simulink model "simulink"  (R2024a)
settings: Solver=ode2  StartTime=0.0  StopTime=100  FixedStep=0.08  RelTol=1e-3  EnableMultiTasking=on
settings Model: Creator=baron  LastModifiedBy=ngoba
settings SolverCC: AlgebraicLoopSolver=TrustRegion
settings DebuggingCC: UnconnectedInputMsg=warning  UnconnectedOutputMsg=warning  UnconnectedLineMsg=warning
settings ModelReferenceCC: EnableRefExpFcnMdlSchedulingChecks=on
settings RTWCC: GPUComputeCapability=3.5

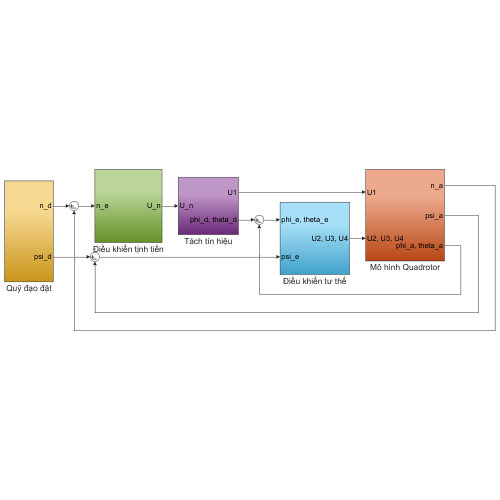
[thumbnail: Simulink's stored preview of the top-level diagram]
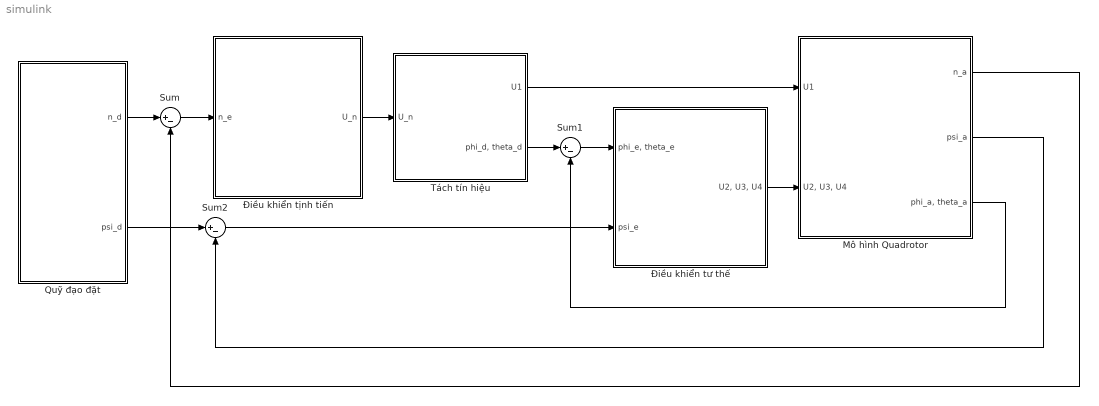
== system simulink ==
  Mô hình Quadrotor : Subsystem
  Quỹ đạo đặt : Subsystem
  Sum : Sum  Inputs=|+-
  Sum1 : Sum  Inputs=|+-
  Sum2 : Sum  Inputs=|+-
  Tách tín hiệu : Subsystem
  Điều khiển tư thế : Subsystem
  Điều khiển tịnh tiến : Subsystem
  wires:
  Sum/1 -> Điều khiển tịnh tiến/1(n_e)
  Quỹ đạo đặt/1(n_d) -> Sum/1
  Điều khiển tịnh tiến/1(U_n) -> Tách tín hiệu/1(U_n)
  Sum1/1 -> Điều khiển tư thế/1("phi_e, theta_e")
  Sum2/1 -> Điều khiển tư thế/2(psi_e)
  Mô hình Quadrotor/1(n_a) -> Sum/2
  Mô hình Quadrotor/2(psi_a) -> Sum2/2
  Mô hình Quadrotor/3("phi_a, theta_a") -> Sum1/2
  Tách tín hiệu/1(U1) -> Mô hình Quadrotor/1(U1)
  Tách tín hiệu/2("phi_d, theta_d") -> Sum1/1
  Điều khiển tư thế/1("U2, U3, U4") -> Mô hình Quadrotor/2("U2, U3, U4")
  Quỹ đạo đặt/2(psi_d) -> Sum2/1

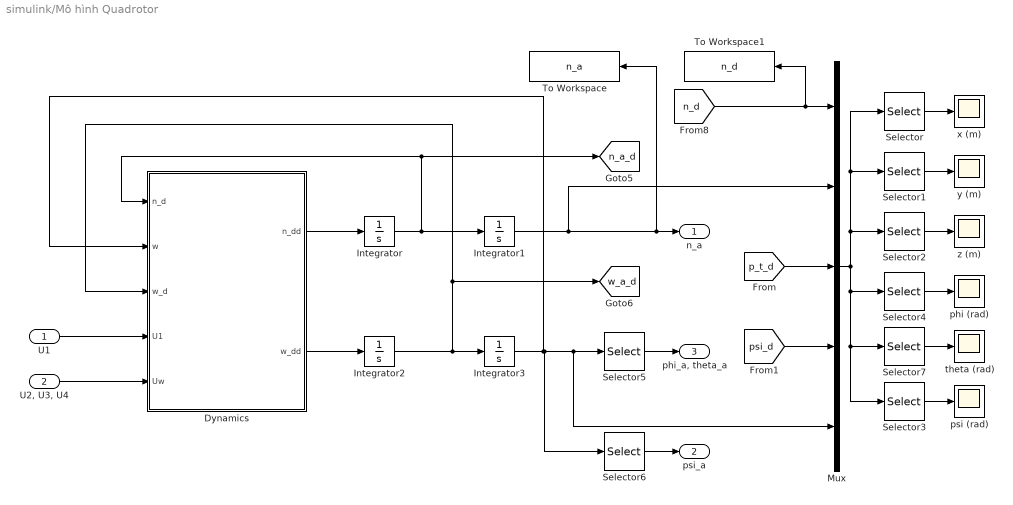
== system simulink/Mô hình Quadrotor ==
  U1 : Inport
  "U2, U3, U4" : Inport  Port=2
  Dynamics : MATLAB Function  TreatAsAtomicUnit=on
  Integrator{,1..3} (4 alike) : Integrator  InitialCondition=[0, 0, 0]'
  Mux : Mux  Inputs=5
  Selector : Selector  InputPortWidth=12  IndexOptions=Index vector (dialog)  Indices=[4 1]  OutputSizes=1
  Selector1 : Selector  InputPortWidth=12  IndexOptions=Index vector (dialog)  Indices=[5 2]  OutputSizes=1
  Selector2 : Selector  InputPortWidth=12  IndexOptions=Index vector (dialog)  Indices=[6 3]  OutputSizes=1
  Selector3 : Selector  InputPortWidth=12  IndexOptions=Index vector (dialog)  Indices=[12 9]  OutputSizes=1
  Selector4 : Selector  InputPortWidth=12  IndexOptions=Index vector (dialog)  Indices=[10 7]  OutputSizes=1
  Selector5 : Selector  InputPortWidth=3  IndexOptions=Index vector (dialog)  Indices=[1 2]  OutputSizes=1
  Selector6 : Selector  InputPortWidth=3  IndexOptions=Index vector (dialog)  Indices=[3]  OutputSizes=1
  Selector7 : Selector  InputPortWidth=12  IndexOptions=Index vector (dialog)  Indices=[11 8]  OutputSizes=1
  To Workspace : ToWorkspace  VariableName=n_a  SampleTime=-1
  To Workspace1 : ToWorkspace  VariableName=n_d  SampleTime=-1
  phi (rad) : Scope
  psi (rad) : Scope
  theta (rad) : Scope
  x (m) : Scope
  y (m) : Scope
  z (m) : Scope
  n_a : Outport
  psi_a : Outport  Port=2
  "phi_a, theta_a" : Outport  Port=3
  tag scope: n_a_d=global, w_a_d=global
  wires:
  Integrator/1 -> Integrator1/1, Dynamics/1(n_d), [n_a_d]
  Integrator3/1 -> Selector6/1, Mux/5, Selector5/1, Dynamics/2(w)
  U1/1 -> Dynamics/4(U1)
  Dynamics/1(n_dd) -> Integrator/1
  Dynamics/2(w_dd) -> Integrator2/1
  "U2, U3, U4"/1 -> Dynamics/5(Uw)
  Integrator2/1 -> Integrator3/1, Dynamics/3(w_d), [w_a_d]
  Selector/1 -> x (m)/1
  [n_d] -> To Workspace1/1, Mux/1
  Selector3/1 -> psi (rad)/1
  Selector1/1 -> y (m)/1
  Selector2/1 -> z (m)/1
  Mux/1 -> Selector2/1, Selector1/1, Selector/1, Selector4/1, Selector7/1, Selector3/1
  Integrator1/1 -> Mux/2, To Workspace/1, n_a/1
  Selector6/1 -> psi_a/1
  Selector5/1 -> "phi_a, theta_a"/1
  Selector4/1 -> phi (rad)/1
  Selector7/1 -> theta (rad)/1
  [p_t_d] -> Mux/3
  [psi_d] -> Mux/4

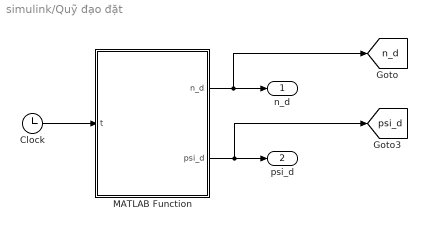
== system simulink/Quỹ đạo đặt ==
  Clock : Clock
  MATLAB Function : MATLAB Function  TreatAsAtomicUnit=on
  n_d : Outport
  psi_d : Outport  Port=2
  tag scope: n_d=global, psi_d=global
  wires:
  Clock/1 -> MATLAB Function/1(t)
  MATLAB Function/1(n_d) -> [n_d], n_d/1
  MATLAB Function/2(psi_d) -> [psi_d], psi_d/1

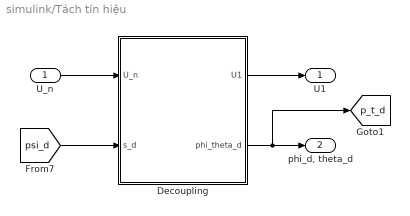
== system simulink/Tách tín hiệu ==
  U_n : Inport
  Decoupling : MATLAB Function  TreatAsAtomicUnit=on
  U1 : Outport
  "phi_d, theta_d" : Outport  Port=2
  tag scope: p_t_d=global
  wires:
  Decoupling/1(U1) -> U1/1
  [psi_d] -> Decoupling/2(s_d)
  U_n/1 -> Decoupling/1(U_n)
  Decoupling/2(phi_theta_d) -> [p_t_d], "phi_d, theta_d"/1

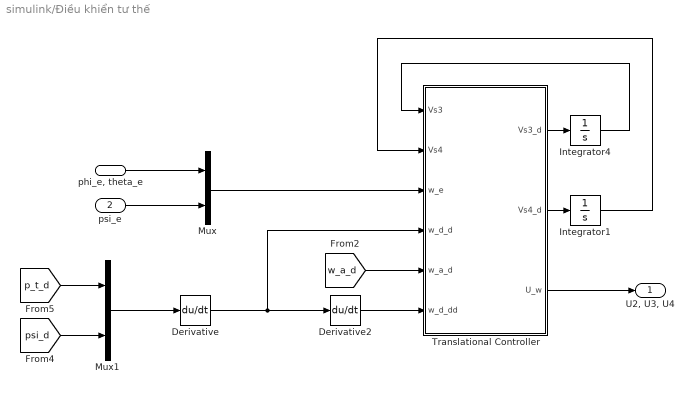
== system simulink/Điều khiển tư thế ==
  "phi_e, theta_e" : Inport
  psi_e : Inport  Port=2
  Derivative : Derivative
  Derivative2 : Derivative
  Integrator1 : Integrator  InitialCondition=[0, 0, 0]'
  Integrator4 : Integrator  InitialCondition=[0, 0, 0]'
  Mux : Mux  Inputs=2
  Mux1 : Mux  Inputs=2
  Translational Controller : MATLAB Function  TreatAsAtomicUnit=on
  "U2, U3, U4" : Outport
  wires:
  Translational Controller/2(Vs4_d) -> Integrator1/1
  Translational Controller/1(Vs3_d) -> Integrator4/1
  [w_a_d] -> Translational Controller/5(w_a_d)
  Derivative2/1 -> Translational Controller/6(w_d_dd)
  Integrator1/1 -> Translational Controller/2(Vs4)
  Translational Controller/3(U_w) -> "U2, U3, U4"/1
  Derivative/1 -> Derivative2/1, Translational Controller/4(w_d_d)
  Integrator4/1 -> Translational Controller/1(Vs3)
  "phi_e, theta_e"/1 -> Mux/1
  psi_e/1 -> Mux/2
  Mux/1 -> Translational Controller/3(w_e)
  Mux1/1 -> Derivative/1
  [psi_d] -> Mux1/2
  [p_t_d] -> Mux1/1

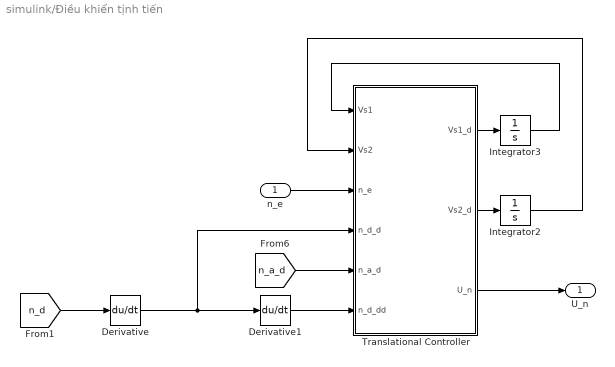
== system simulink/Điều khiển tịnh tiến ==
  n_e : Inport
  Derivative : Derivative
  Derivative1 : Derivative
  Integrator2 : Integrator  InitialCondition=[0, 0, 0]'
  Integrator3 : Integrator  InitialCondition=[0, 0, 0]'
  Translational Controller : MATLAB Function  TreatAsAtomicUnit=on
  U_n : Outport
  wires:
  [n_d] -> Derivative/1
  Derivative/1 -> Translational Controller/4(n_d_d), Derivative1/1
  Translational Controller/3(U_n) -> U_n/1
  Translational Controller/1(Vs1_d) -> Integrator3/1
  Integrator3/1 -> Translational Controller/1(Vs1)
  Translational Controller/2(Vs2_d) -> Integrator2/1
  Integrator2/1 -> Translational Controller/2(Vs2)
  n_e/1 -> Translational Controller/3(n_e)
  Derivative1/1 -> Translational Controller/6(n_d_dd)
  [n_a_d] -> Translational Controller/5(n_a_d)

== matlab function simulink/Mô hình Quadrotor/Dynamics ==
  settings: updateMethod=DISCRETE
  data: n_d input; n_dd output; w_dd output; w input; w_d input; U1 input; Uw input
function [n_dd, w_dd] = fcn(n_d, w, w_d, U1, Uw)
    % Parameters
    m = 0.486;
    g = 9.810;
    Mm = diag([m, m, m]);
    Gg = [0, 0, -m*g]';
    l = diag([0.250, 0.250, 1]);
    I = diag([4.856e-3, 4.856e-3, 8.801e-3]);
    cdn = diag([5.560e-4, 5.560e-4, 6.350e-4]);
    kdn = diag([1e-4, 1e-4, 1e-4]);
    kp = 3.230e-7;
    kd = 2.980e-5;
    W_to_U = [ kd,  kd, kd,  kd;
                0,  kd,  0, -kd;
              -kd,   0, kd,   0;
               kp, -kp, kp, -kp];
    Ir = diag([5e-5, 5e-5, 5e-5]);
    % Translational function
    FD = -cdn*n_d;   
    % Rotational function
    W = sqrt((W_to_U^-1)*[U1; Uw]);
    W_ = diag([W(1)-W(2)+W(3)-W(4), W(1)-W(2)+W(3)-W(4), W(1)-W(2)+W(3)-W(4)]);
    Gf = kdn*(w.^2);
    tM = Ir*W_*[w(2), w(1), 0]';
    % Disturbances
    n_dis = 4*(rand(3, 1) - 0.5);
    w_dis = [2*(rand(2, 1) - 0.5); 0.5*(rand - 0.5)];
    % Translational dynamics
    F = [0, 0, U1]';
    Jr = R_M(w(1), w(2), w(3));
    n_dd = (Mm^-1)*(Jr*F + Gg + FD) + n_dis;
    % Rotational dynamics
    tC = l*Uw;
    w_dd = (I^-1)*(cross(-w_d, I*w_d) + Gf + tM + tC) + w_dis;
end
% Rotation matrix
function Jr = R_M(phi, theta, psi)
    Jr = [0, 0, cos(phi)*cos(psi)*sin(theta) + sin(phi)*sin(psi);
          0, 0, cos(phi)*sin(psi)*sin(theta) - sin(phi)*cos(psi);
          0, 0, cos(phi)*cos(theta)                             ];
end

== matlab function simulink/Điều khiển tịnh tiến/Translational Controller ==
  data: Vs1 input; Vs2 input; Vs1_d output; Vs2_d output; n_e input; n_d_d input; n_a_d input; U_n output; n_d_dd input
function [Vs1_d, Vs2_d, U_n] = fcn(Vs1, Vs2, n_e, n_d_d, n_a_d, n_d_dd)
    A1 = diag([1, 1, 1]);
    B1 = diag([2, 2, 2]);
    Vs1_d = -(A1 + abs(diag(n_e)))*Vs1 + B1*n_e;
    
    A2 = diag([4, 4, 4]);
    B2 = diag([8, 8, 8]);
    K1 = diag([0.1, 0.1, 0.1]);
    n_ev = n_d_d + K1*Vs1 - n_a_d;
    Vs2_d = -(A2 + abs(diag(n_ev)))*Vs2 + B2*n_ev;

    K2 = diag([1, 1, 1]);
    f_n = [0, 0, 0]';
    U_n = n_d_dd - f_n + K1*Vs1_d + n_e + K2*Vs2;
end

== matlab function simulink/Tách tín hiệu/Decoupling ==
  data: U_n input; U1 output; s_d input; phi_theta_d output
function [U1, phi_theta_d] = fcn(U_n, s_d)
    m = 0.486;
    g = 9.810;
    t_d = atan((U_n(1)*cos(s_d) + U_n(2)*sin(s_d))/(U_n(3) + g));
    p_d = atan(cos(t_d)*(U_n(1)*sin(s_d) - U_n(2)*cos(s_d))/(U_n(3) + g));
    phi_theta_d = [p_d, t_d]';
    U1 = m*sqrt(U_n(1)^2 + U_n(2)^2 + (U_n(3) + g)^2);
end

== matlab function simulink/Quỹ đạo đặt/MATLAB Function ==
  data: t input; n_d output; psi_d output
function [n_d, psi_d] = fcn(t)
    n_d = [1 + 8*sin(0.1*t - pi/4), -8 + 8*cos(0.1*t - pi/4), 2 + 0.2*t]';
    psi_d = 0;
end

== matlab function simulink/Điều khiển tư thế/Translational Controller ==
  data: Vs3 input; Vs4 input; Vs3_d output; Vs4_d output; w_e input; w_d_d input; w_a_d input; U_w output; w_d_dd input
function [Vs3_d, Vs4_d, U_w] = fcn(Vs3, Vs4, w_e, w_d_d, w_a_d, w_d_dd)
    A3 = diag([5, 5, 5]);
    B3 = diag([1, 1, 1]);
    Vs3_d = -(A3 + abs(diag(w_e)))*Vs3 + B3*w_e;
    
    A4 = diag([2, 2, 2]);
    B4 = diag([10, 10, 10]);
    K3 = diag([3, 3, 3]);
    n_eu = w_d_d + K3*Vs3 - w_a_d;
    Vs4_d = -(A4 + abs(diag(n_eu)))*Vs4 + B4*n_eu;

    K4 = diag([5, 5, 5]);
    w_d_dd1 = [0, 0, w_d_dd(3)]';
    I = diag([4.856e-3, 4.856e-3, 8.801e-3]);
    f_w = cross(-w_a_d, I*w_a_d);
    l = diag([0.250, 0.250, 1]);
    U_w = (I/l)*(w_d_dd1 - f_w + K3*Vs3_d + w_e + K4*Vs4);
end
